simulink model "feedback_plant"  (R2020b)
settings: Solver=FixedStepDiscrete  StartTime=0.0  StopTime=inf  FixedStep=T_sample_control  MaxStep=0.1  RelTol=1e-3  EnableMultiTasking=on
settings Model: DataDictionary=pid.sldd  ModifiedByFormat=The MathWorks Inc.  Creator=The MathWorks, Inc.  LastModifiedBy=The MathWorks Inc.
settings DataIOCC: SaveFormat=Array  ReturnWorkspaceOutputs=off
settings OptimizationCC: DefaultParameterBehavior=Inlined  ExpressionDepthLimit=2147483647  LifeSpan=1
settings DebuggingCC: UnderspecifiedInitializationDetection=Classic  MergeDetectMultiDrivingBlocksExec=none  SolverPrmCheckMsg=warning  FcnCallInpInsideContextMsg=warning  AllowSymbolicDim=off  StateNameClashWarn=warning  SFUnexpectedBacktrackingDiag=warning  SFNoUnconditionalDefaultTransitionDiag=warning  SFExecutionAtInitializationDiag=none  ArithmeticOperatorsInVariantConditions=warning
settings HardwareCC: ProdBitPerPointer=32  ProdBitPerSizeT=32  ProdBitPerPtrDiffT=32  ProdLargestAtomicFloat=None  ProdIntDivRoundTo=Undefined  ProdEndianess=Unspecified  ProdWordSize=32  ProdHWDeviceType=32-bit Generic
settings ModelReferenceCC: PropagateSignalLabelsOutOfModel=off
settings SFSimCC: SimUseLocalCustomCode=off  CustomCodeUndefinedFunction=UseInterfaceOnly
settings RTWCC: RTWUseLocalCustomCode=off
settings CodeAppCC: StateflowObjectComments=on
settings GRTTargetCC: TargetLangStandard=C89/C90 (ANSI)  CombineOutputUpdateFcns=off  GRTInterface=on
settings ConfigComp: CovMetricSettings=dw  CovSaveCumulativeToWorkspaceVar=on  CovSaveSingleToWorkspaceVar=on  CovExternalEMLEnable=off  CovSFcnEnable=off

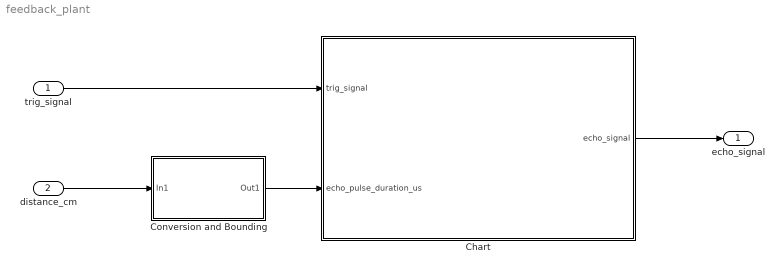
== system feedback_plant ==
  trig_signal : Inport  OutDataTypeStr=boolean
  distance_cm : Inport  Port=2
  Chart : Stateflow chart  TreatAsAtomicUnit=on
  Conversion and Bounding : Subsystem
  echo_signal : Outport  OutDataTypeStr=boolean
  wires:
  trig_signal/1 -> Chart/1(trig_signal)
  Chart/1(echo_signal) -> echo_signal/1
  distance_cm/1 -> Conversion and Bounding/1(In1)
  Conversion and Bounding/1(Out1) -> Chart/2(echo_pulse_duration_us)

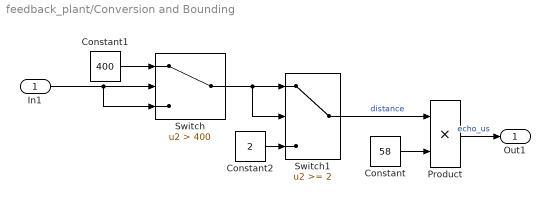
== system feedback_plant/Conversion and Bounding ==
  In1 : Inport
  Constant : Constant  Value=58
  Constant1 : Constant  Value=400
  Constant2 : Constant  Value=2
  Product : Product
  Switch : Switch  Criteria=u2 > Threshold  Threshold=400
  Switch1 : Switch  Threshold=2
  Out1 : Outport
  wires:
  Constant1/1 -> Switch/1
  Constant2/1 -> Switch1/3
  Switch/1 -> Switch1/2, Switch1/1
  Constant/1 -> Product/2
  In1/1 -> Switch/3, Switch/2
  Product/1 -> Out1/1  "echo_us"
  Switch1/1 -> Product/1  "distance"

== stateflow chart feedback_plant/Chart ==
  state WAIT_TO_RISE
  state WAIT_TO_FALL
  state RESPONS_ECHO_SIGNAL
    entry:
    echo_signal = true;
    exit:
    echo_signal = false;
  (default) -> WAIT_TO_RISE
  (junction 16) -> WAIT_TO_RISE
  (junction 22) -> (junction 16)
  WAIT_TO_RISE -> WAIT_TO_FALL : [trig_signal == true]
  WAIT_TO_FALL -> (junction 22) [order 1] : [trig_signal == false]
  (junction 14) -> (junction 22)
  WAIT_TO_FALL -> RESPONS_ECHO_SIGNAL [order 2] : [after(10,usec)]
  RESPONS_ECHO_SIGNAL -> (junction 14) : after(echo_pulse_duration_us, usec)
  data: trig_signal input boolean; echo_pulse_duration_us input double; echo_signal output boolean
